simulink library "dlbsBlockReciprocal"  (R2025b)
settings: Solver=VariableStepAuto  StartTime=0.0  StopTime=10.0  RelTol=1e-3
libraries: dlbsBlockExtractGradientGF x1, dlbsBlockInsertGradientGF x1
settings Model: Creator=lt6037  LastModifiedBy=lt6037

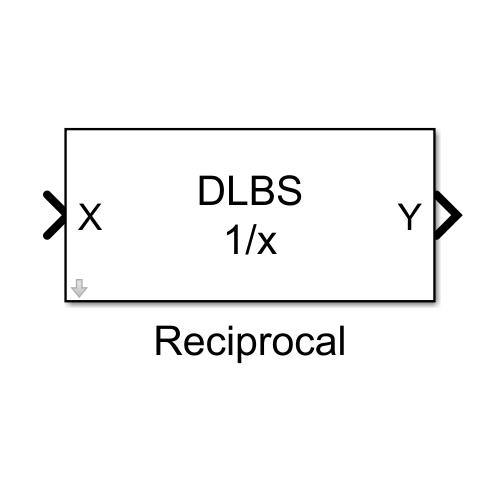
[thumbnail: Simulink's stored preview of the top-level diagram]
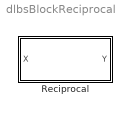
== system dlbsBlockReciprocal ==
  Reciprocal : Subsystem
      mask help: Computes the reciprocal of the input tensor. The operation is applied element-wise across all tensor elements.
      mask Help: web("dlbsHelpBlockReciprocal.html")
      mask Display: fprintf("DLBS\n1/x")

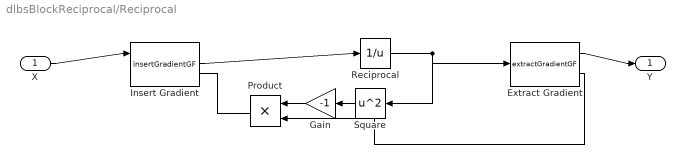
== system dlbsBlockReciprocal/Reciprocal ==
  X : Inport
  Extract Gradient : dlbsBlockExtractGradientGF/extractGradientGF
  Gain : Gain  Gain=-1
  Insert Gradient : dlbsBlockInsertGradientGF/insertGradientGF
  Product : Product
  Reciprocal : Math  Operator=reciprocal
  Square : Math  Operator=square
  Y : Outport
  wires:
  Extract Gradient/2 -> Product/2
  Product/1 -> Insert Gradient/2
  Insert Gradient/1 -> Reciprocal/1
  Reciprocal/1 -> Extract Gradient/1, Square/1
  Gain/1 -> Product/1
  Square/1 -> Gain/1
  Extract Gradient/1 -> Y/1
  X/1 -> Insert Gradient/1
